simulink model "HYBVS"  (Simulink 5.0)
settings: Solver=ode45  StartTime=0.0  StopTime=30.0  RelTol=1e-3
values from neighbouring files (symbols this model uses):
  c = camera(1000,1000,256,256,512,512)    [initHBVS.m]    (also in pose0.mat = ; pose1.mat = ; sim1.mat = ; task_endeff.mat = )
  p = reshape(u,2,n)    [CamView.m]    (also in initHBVS.m = polyhedra([0.0 0.0 0; 0.25 0.25 0; -0.25 0.25 0; -0.25 -0.25; pose0.mat = ; pose1.mat = ; sim1.mat = )
  T0c_0 = T0c    [initHBVS.m]    (also in sim1.mat = )
  T0c_x = T0c    [initHBVS.m]    (also in sim1.mat = )
  T0o =     [pose0.mat]    (also in pose1.mat; sim1.mat; task_endeff.mat; task_stereo.mat)
undefined symbols (not defined in the file or in its folder): coords, get, GetHMatrix
libraries: vs x12
settings Model: LastModifiedBy=ecervera  BooleanDataType=off

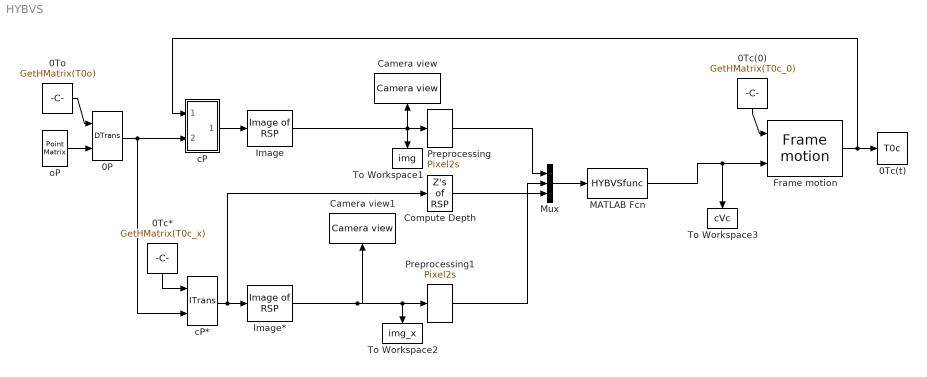
== system HYBVS ==
  0P : vs/Features/DTrans  SimViewingDevice=off  DataTypeOverride=UseLocalSettings  MinMaxOverflowLogging=UseLocalSettings
      settings: Permissions=ReadWrite  RTWFcnNameOpts=Auto  RTWFileNameOpts=Auto
  0Tc(0) : Constant  Orientation=down  Value=GetHMatrix(T0c_0)  VectorParams1D=off
  0Tc(t) : ToWorkspace  VariableName=T0c  SampleTime=-1  SaveFormat=StructureWithTime
  0Tc* : Constant  Orientation=down  Value=GetHMatrix(T0c_x)  VectorParams1D=off
  0To : Constant  Value=GetHMatrix(T0o)  VectorParams1D=off
  Camera view : vs/Camera/Camera view  Orientation=up  ms=15  em=normal  umin=0  umax=get(c,'hres')-1  vmin=0  vmax=get(c,'vres')-1  st=-1
  Camera view1 : vs/Camera/Camera view  Orientation=up  ms=15  em=normal  umin=0  umax=get(c,'hres')-1  vmin=0  vmax=get(c,'vres')-1  st=-1
  Compute Depth : vs/Features/Z's of RSP  SimViewingDevice=off  DataTypeOverride=UseLocalSettings  MinMaxOverflowLogging=UseLocalSettings
      settings: Permissions=ReadWrite  RTWFcnNameOpts=Auto  RTWFileNameOpts=Auto
  Frame motion : vs/Pose/Frame motion  SimViewingDevice=off  DataTypeOverride=UseLocalSettings  MinMaxOverflowLogging=UseLocalSettings
      settings: Permissions=ReadWrite  RTWFcnNameOpts=Auto  RTWFileNameOpts=Auto
  Image : vs/Camera/Image of RSP  fu=get(c,'fu')  fv=get(c,'fv')  u0=get(c,'u0')  v0=get(c,'v0')
  Image* : vs/Camera/Image of RSP  fu=get(c,'fu')  fv=get(c,'fv')  u0=get(c,'u0')  v0=get(c,'v0')
  MATLAB Fcn : MATLABFcn  MATLABFcn=HYBVSfunc  OutputDimensions=[6 1]  Output1D=off
  Mux : Mux  Inputs=3
  Preprocessing : vs/Jacobian/Pixel2s  fu=get(c,'fu')  fv=get(c,'fv')  u0=get(c,'u0')  v0=get(c,'v0')
  Preprocessing1 : vs/Jacobian/Pixel2s  fu=get(c,'fu')  fv=get(c,'fv')  u0=get(c,'u0')  v0=get(c,'v0')
  To Workspace1 : ToWorkspace  VariableName=img  SampleTime=-1  SaveFormat=StructureWithTime
      settings: Orientation=down
  To Workspace2 : ToWorkspace  VariableName=img_x  SampleTime=-1  SaveFormat=StructureWithTime
      settings: Orientation=down
  To Workspace3 : ToWorkspace  VariableName=cVc  SampleTime=-1  SaveFormat=StructureWithTime
      settings: Orientation=down
  cP : Subsystem  AncestorBlock=vs/Features/ITrans
  cP* : vs/Features/ITrans  SimViewingDevice=off  DataTypeOverride=UseLocalSettings  MinMaxOverflowLogging=UseLocalSettings
      settings: Permissions=ReadWrite  RTWFcnNameOpts=Auto  RTWFileNameOpts=Auto
  oP : vs/Features/Point Matrix  m=coords(p)
  wires:
  oP/1 -> 0P/2
  cP/1(bP) -> Image/1
  Image/1 -> Camera view/1, Preprocessing/1, To Workspace1/1
  Preprocessing/1 -> Mux/1
  Compute Depth/1 -> Mux/3
  Frame motion/1 -> 0Tc(t)/1, cP/1(aTb)
  0Tc*/1 -> cP*/1
  cP*/1 -> Image*/1, Compute Depth/1
  0Tc(0)/1 -> Frame motion/1
  0To/1 -> 0P/1
  0P/1 -> cP/2(aP), cP*/2
  MATLAB Fcn/1 -> Frame motion/2, To Workspace3/1
  Image*/1 -> Preprocessing1/1, To Workspace2/1, Camera view1/1
  Preprocessing1/1 -> Mux/2
  Mux/1 -> MATLAB Fcn/1

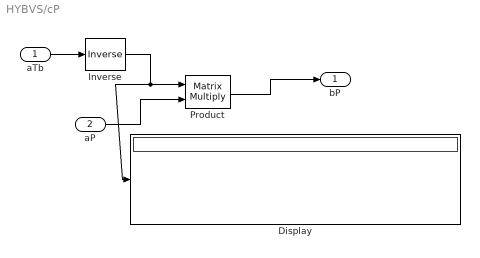
== system HYBVS/cP ==
  aTb : Inport
  aP : Inport  Port=2
  Display : Display
  Inverse : vs/Pose/Inverse  SimViewingDevice=off  DataTypeOverride=UseLocalSettings  MinMaxOverflowLogging=UseLocalSettings
      settings: Permissions=ReadWrite  RTWFcnNameOpts=Auto  RTWFileNameOpts=Auto
  Product : Product  Multiplication=Matrix(*)  SaturateOnIntegerOverflow=on  InputSameDT=on
  bP : Outport
  wires:
  Inverse/1 -> Product/1, Display/1
  aTb/1 -> Inverse/1
  Product/1 -> bP/1
  aP/1 -> Product/2
